simulink model "Temp_Protection_Testing"  (R2024a)
settings: Solver=FixedStepAuto  StartTime=0.0  StopTime=10.0  FixedStep=0.1  RelTol=1e-3
settings Model: Creator=gopin  LastModifiedBy=gopin
settings OptimizationCC: DefaultParameterBehavior=Inlined  EnhancedBackFolding=on  PassReuseOutputArgsAs=Individual arguments  ZeroExternalMemoryAtStartup=off  ZeroInternalMemoryAtStartup=off  OptimizeBlockOrder=speed  DifferentSizesBufferReuse=on  OptimizationCustomize=off  EfficientTunableParamExpr=on
settings DebuggingCC: ParameterTunabilityLossMsg=error
settings SFSimCC: MATLABDynamicMemAlloc=off
settings RTWCC: Description=Embedded Coder  SystemTargetFile=ert.tlc  TemplateMakefile=ert_default_tmf
settings CodeAppCC: ForceParamTrailComments=on  IgnoreCustomStorageClasses=off  OperatorAnnotations=on  SimulinkDataObjDesc=on  SFDataObjDesc=on  InsertBlockDesc=on
settings ERTTargetCC: TargetLangStandard=C99 (ISO)  GenerateSampleERTMain=on  InlinedParameterPlacement=NonHierarchical  ERTCustomFileTemplate=example_file_process.tlc

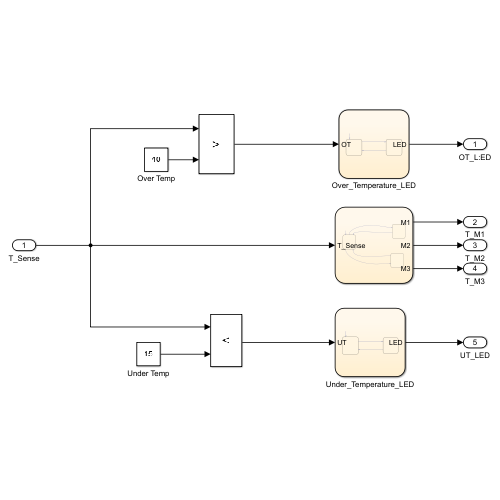
[thumbnail: Simulink's stored preview of the top-level diagram]
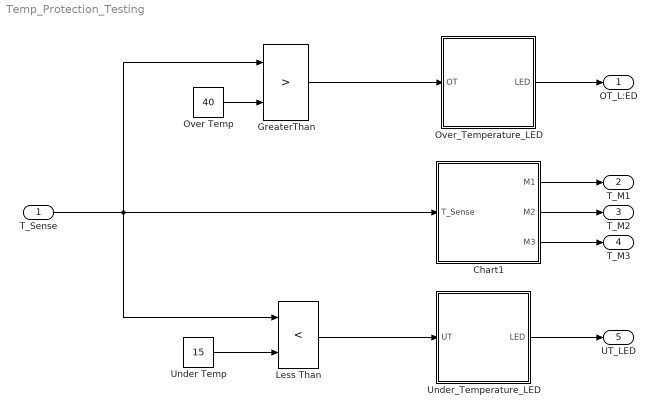
== system Temp_Protection_Testing ==
  T_Sense : Inport
  Chart1 : Stateflow chart  TreatAsAtomicUnit=on
      settings: PortSchema="{\"entries\":[{\"content\":{\"sides\":[{\"content\":{\"connectorIds\":[\"In1\"]},\"type\":\"ConnectorPlacement.EquallySpacedRectSide\",\"uuid\":\"05ea740b-acd1-442a-a5fc-8d5534125df7\"},{\"content\":{\"connectorIds\":[\"Out1\",\"Out3\",\"Out2\"],\"side\":\"RIGHT\"},\"type\":\"ConnectorPlacement.EquallySpacedRectSide\",\"uuid\":\"8a7de145-2aa2-4311-b5d6-9482723dc71b\"},{\"content\":{\"side\":\"TOP\"},\"type\":\"ConnectorPlacement.EquallySpacedRectSide\",\"uuid\":\"63b1bd07-fd81-4427-8db4-3d8b6b536b2e\"}]},\"type\":\"ConnectorPlacement.EquallySpacedConnector\",\"uuid\":\"2e40ebd9-6121-4c1e-a234-5e0461cc6cd1\"}],\"packageUris\":[\"http://schema.mathworks.com/mf0/Connector/R2020b\"],\"version\":\"1.0\"}"
  GreaterThan : RelationalOperator  Operator=>  OutDataTypeStr=boolean  RndMeth=Simplest  InputSameDT=off
  Less Than : RelationalOperator  Operator=<  OutDataTypeStr=boolean  RndMeth=Simplest  InputSameDT=off
  Over Temp : Constant  Value=40
  Over_Temperature_LED : Stateflow chart  TreatAsAtomicUnit=on
  Under Temp : Constant  Value=15
  Under_Temperature_LED : Stateflow chart  TreatAsAtomicUnit=on
  OT_L:ED : Outport
  T_M1 : Outport  Port=2
  T_M2 : Outport  Port=3
  T_M3 : Outport  Port=4
  UT_LED : Outport  Port=5
  wires:
  Chart1/1(M1) -> T_M1/1
  Under_Temperature_LED/1(LED) -> UT_LED/1
  Over_Temperature_LED/1(LED) -> OT_L:ED/1
  Chart1/2(M3) -> T_M3/1
  T_Sense/1 -> GreaterThan/1, Chart1/1(T_Sense), Less Than/1
  Chart1/3(M2) -> T_M2/1
  Under Temp/1 -> Less Than/2
  Less Than/1 -> Under_Temperature_LED/1(UT)
  GreaterThan/1 -> Over_Temperature_LED/1(OT)
  Over Temp/1 -> GreaterThan/2

== stateflow chart Temp_Protection_Testing/Over_Temperature_LED ==
  state LED_OFF
    en:
    LED=0;
    du:
    LED=0;
  state LED_ON
    en:
    LED=1;
  (default) -> LED_OFF
  LED_OFF -> LED_ON : [OT==1]
  LED_ON -> LED_OFF : [OT==0]
  data: LED output; OT input

== stateflow chart Temp_Protection_Testing/Chart1 ==
  state OT_Cutoff
    en:
    M1=0;
    M2=0;
    M3=0;
  state Initial_Start
    en:
    M1=1;
    M2=1;
    M3=1;
  state UT_Cutoff
    en:
    M1=0;
    M2=0;
    M3=0;
  Initial_Start -> OT_Cutoff [order 1] : [T_Sense>40]
  (default) -> Initial_Start
  OT_Cutoff -> Initial_Start : [T_Sense<35 && after(10,sec)]
  Initial_Start -> UT_Cutoff [order 2] : [T_Sense<15]
  UT_Cutoff -> Initial_Start : [T_Sense>15 && after(10,sec)]
  data: M1 output; M3 output; M2 output; T_Sense input

== stateflow chart Temp_Protection_Testing/Under_Temperature_LED ==
  state LED_OFF
    en:
    LED=0;
    du:
    LED=0;
  state LED_ON
    en:
    LED=1;
  (default) -> LED_OFF
  LED_OFF -> LED_ON : [UT==1]
  LED_ON -> LED_OFF : [UT==0]
  data: UT input; LED output
